simulink model "Arranque_2M"  (R2018b)
settings: Solver=VariableStepAuto  StartTime=0.0  StopTime=32  MaxStep=1e-4  RelTol=1e-3
libraries: powerlib x24, powerlib_meascontrol x12
settings Model: Creator=Guille2  LastModifiedBy=grbos
settings SFSimCC: SimUseLocalCustomCode=off
settings RTWCC: RTWUseLocalCustomCode=off

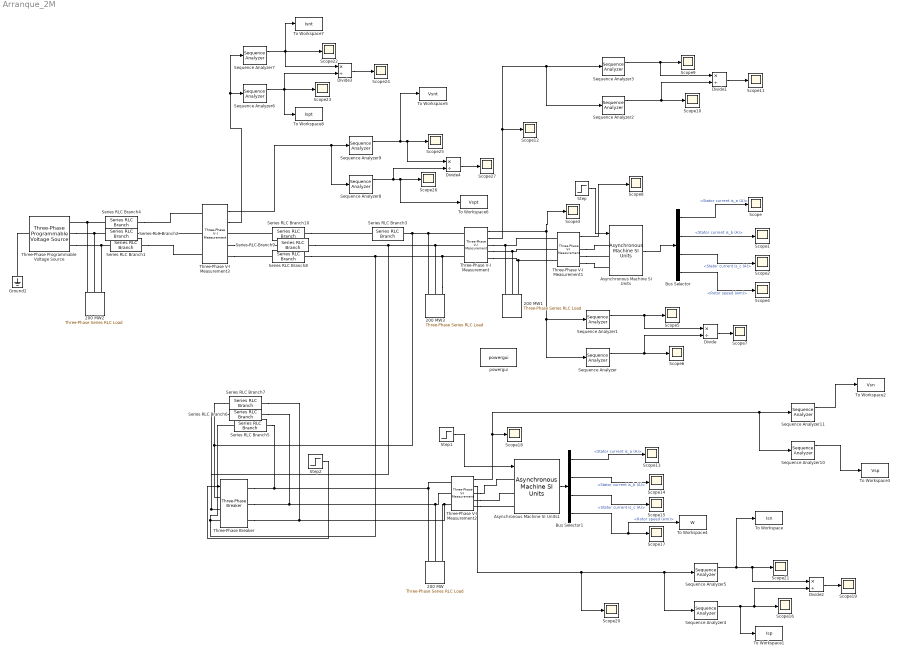
== system Arranque_2M ==
  200 MW{,1..3} (4 alike) : powerlib/Elements/Three-Phase Series RLC Load  LConnTagsString=A|B|C  Configuration=Y (grounded)  NominalVoltage=380  Vabc=[1e3 1e3 1e3]  Vabcp=[1e3 1e3 1e3]  NominalFrequency=50  UnbalancedPower=off  ActivePower=2  InductivePower=0  CapacitivePower=0  Pabc=[10e3 9e3 11e3]  QLabc=[100 90 110]  QCabc=[100 90 110]  Pabcp=[10e3 9e3 11e3]  QLabcp=[100 90 110]  QCabcp=[100 90 110]  Measurements=None  LoadType=constant Z
      settings: SourceProductName=Simscape Electrical
  Asynchronous Machine SI Units : powerlib/Machines/Asynchronous Machine SI Units  RotorType=Squirrel-cage  PresetModel=No  MechanicalLoad=Torque Tm  ShowDetailedParameters=on  ReferenceFrame=Stationary  Units=SI  MeasurementBus=off  NominalParameters=[1.6e+05 400 50]  Stator=[0.01379 0.000152]  Rotor=[0.01728 0.000252]  Cage1=[0.4155 0.002066]  Cage2=[0.4168 0.0003495]  Lm=0.00769  Mechanical=[10 0.05658 1]  PolePairs=2  InitialConditions=[1 0 0 0 0 0 0 0]  SimulateSaturation=off  Saturation=[14.03593122, 27.81365428, 53.79336849, 72.68890987, 97.98006896, 148.6815601, 215.7428561, 302.9841135, 428.7778367 ; 230, 322, 414, 460, 506, 552, 598, 644, 690]  LoadFlowParameters=1492000  TsPowergui=0  TsBlock=-1  IterativeModel=Trapezoidal non iterative  IterativeDiscreteModel=Trapezoidal non iterative  Pmec=1.492e+006
      settings: SourceProductName=Simscape Electrical
  Asynchronous Machine SI Units1 : powerlib/Machines/Asynchronous Machine SI Units  RotorType=Squirrel-cage  PresetModel=No  MechanicalLoad=Torque Tm  ShowDetailedParameters=on  ReferenceFrame=Stationary  Units=SI  MeasurementBus=off  NominalParameters=[1.6e+05 400 50]  Stator=[0.01379 0.000152]  Rotor=[0.01728 0.000252]  Cage1=[0.4155 0.002066]  Cage2=[0.4168 0.0003495]  Lm=0.00769  Mechanical=[10 0.05658 1]  PolePairs=2  InitialConditions=[1 0 0 0 0 0 0 0]  SimulateSaturation=off  Saturation=[14.03593122, 27.81365428, 53.79336849, 72.68890987, 97.98006896, 148.6815601, 215.7428561, 302.9841135, 428.7778367 ; 230, 322, 414, 460, 506, 552, 598, 644, 690]  LoadFlowParameters=1492000  TsPowergui=0  TsBlock=-1  IterativeModel=Trapezoidal non iterative  IterativeDiscreteModel=Trapezoidal non iterative  Pmec=1.492e+006
      settings: SourceProductName=Simscape Electrical
  Bus Selector : BusSelector  OutputSignals=Stator measurements.Stator current is_a (A),Stator measurements.Stator current is_b (A),Stator measurements.Stator current is_c (A),Mechanical.Rotor speed (wm)
  Bus Selector1 : BusSelector  OutputSignals=Stator measurements.Stator current is_a (A),Stator measurements.Stator current is_b (A),Stator measurements.Stator current is_c (A),Mechanical.Rotor speed (wm)
  Divide{,1..4} (5 alike) : Product  Inputs=*/
  Ground2 : powerlib/Elements/Ground  LConnTagsString=a
      settings: SourceProductName=Simscape Electrical
  Scope{,1..27} (28 alike) : Scope
  Sequence Analyzer{,2,4,6,8,10} (6 alike) : powerlib_meascontrol/Measurements/Sequence Analyzer  Freq=50  n=1  seq=Positive  InInit=[1, 0]  Ts=0
      settings: SourceProductName=Simscape Electrical  SourceProductBaseCode=PS
  Sequence Analyzer{1,3,5,7,9,11} (6 alike) : powerlib_meascontrol/Measurements/Sequence Analyzer  Freq=50  n=1  seq=Negative  InInit=[1, 0]  Ts=0
      settings: SourceProductName=Simscape Electrical  SourceProductBaseCode=PS
  Series RLC Branch{1..4} (4 alike) : powerlib/Elements/Series RLC Branch  LConnTagsString=__new0  RConnTagsString=__new0  BranchType=R  Resistance=0.01  Inductance=1.0  SetiL0=off  InitialCurrent=0  Capacitance=1.0  Setx0=off  InitialVoltage=0  Measurements=None
      settings: SourceProductName=Simscape Electrical
  Series RLC Branch10 : powerlib/Elements/Series RLC Branch  LConnTagsString=__new0  RConnTagsString=__new0  BranchType=R  Resistance=0.02  Inductance=1.0  SetiL0=off  InitialCurrent=0  Capacitance=1.0  Setx0=off  InitialVoltage=0  Measurements=None
      settings: SourceProductName=Simscape Electrical
  Series RLC Branch5 : powerlib/Elements/Series RLC Branch  LConnTagsString=__new0  RConnTagsString=__new0  BranchType=R  Resistance=300  Inductance=1.0  SetiL0=off  InitialCurrent=0  Capacitance=1.0  Setx0=off  InitialVoltage=0  Measurements=None
      settings: SourceProductName=Simscape Electrical
  Series RLC Branch6 : powerlib/Elements/Series RLC Branch  LConnTagsString=__new0  RConnTagsString=__new0  BranchType=R  Resistance=300  Inductance=1.0  SetiL0=off  InitialCurrent=0  Capacitance=1.0  Setx0=off  InitialVoltage=0  Measurements=None
      settings: SourceProductName=Simscape Electrical
  Series RLC Branch7 : powerlib/Elements/Series RLC Branch  LConnTagsString=__new0  RConnTagsString=__new0  BranchType=R  Resistance=300  Inductance=1.0  SetiL0=off  InitialCurrent=0  Capacitance=1.0  Setx0=off  InitialVoltage=0  Measurements=None
      settings: SourceProductName=Simscape Electrical
  Series RLC Branch8 : powerlib/Elements/Series RLC Branch  LConnTagsString=__new0  RConnTagsString=__new0  BranchType=R  Resistance=0.02  Inductance=1.0  SetiL0=off  InitialCurrent=0  Capacitance=1.0  Setx0=off  InitialVoltage=0  Measurements=None
      settings: SourceProductName=Simscape Electrical
  Series RLC Branch9 : powerlib/Elements/Series RLC Branch  LConnTagsString=__new0  RConnTagsString=__new0  BranchType=R  Resistance=0.02  Inductance=1.0  SetiL0=off  InitialCurrent=0  Capacitance=1.0  Setx0=off  InitialVoltage=0  Measurements=None
      settings: SourceProductName=Simscape Electrical
  Step : Step  Time=8  After=500  SampleTime=0
  Step1 : Step  Time=24  After=500  SampleTime=0
  Step2 : Step  Time=16  SampleTime=0
  Three-Phase Programmable Voltage Source : powerlib/Electrical Sources/Three-Phase Programmable Voltage Source  PositiveSequence="[380  0 50]"  VariationEntity=None  VariationType=Table of time-amplitude pairs  VariationTypeAlt=Step  VariationStep=0.5  VariationRate=10  VariationMagnitude=0.3  VariationFrequency=2  VariationTiming=[1 2]  VariationPhaseA=off  Amplitudes=[1 0.8 1.2 1.0]  TimeValues=[0 0.1 0.15 0.2]  HarmonicGeneration=off  HarmonicA=[1 0.73 0 1]  HarmonicB=[0 0 0 0]  Timing="[8  16]"  BusType=swing  Pref=0  Qref=0  Qmin=-inf  Qmax=inf
      settings: SourceProductName=Simscape Electrical
  Three-Phase V-I Measurement : powerlib/Measurements/Three-Phase V-I Measurement  VoltageMeasurement=phase-to-ground  SetLabelV=off  LabelV=Vabc  Vpu=off  VpuLL=off  CurrentMeasurement=yes  SetLabelI=off  LabelI=Iabc  Ipu=off  Pbase=100e6  Vbase=500e3  OutputType=Complex  PhasorSimulation=off  PSBequivalent=0
      settings: SourceProductName=Simscape Electrical
  Three-Phase V-I Measurement1 : powerlib/Measurements/Three-Phase V-I Measurement  VoltageMeasurement=phase-to-phase  SetLabelV=off  LabelV=Vabc  Vpu=off  VpuLL=off  CurrentMeasurement=yes  SetLabelI=off  LabelI=Iabc  Ipu=off  Pbase=100e6  Vbase=500e3  OutputType=Complex  PhasorSimulation=off  PSBequivalent=0
      settings: SourceProductName=Simscape Electrical
  Three-Phase V-I Measurement2 : powerlib/Measurements/Three-Phase V-I Measurement  VoltageMeasurement=phase-to-ground  SetLabelV=off  LabelV=Vabc  Vpu=off  VpuLL=off  CurrentMeasurement=yes  SetLabelI=off  LabelI=Iabc  Ipu=off  Pbase=100e6  Vbase=500e3  OutputType=Complex  PhasorSimulation=off  PSBequivalent=0
      settings: SourceProductName=Simscape Electrical
  Three-Phase V-I Measurement3 : powerlib/Measurements/Three-Phase V-I Measurement  VoltageMeasurement=phase-to-ground  SetLabelV=off  LabelV=Vabc  Vpu=off  VpuLL=off  CurrentMeasurement=yes  SetLabelI=off  LabelI=Iabc  Ipu=off  Pbase=100e6  Vbase=500e3  OutputType=Complex  PhasorSimulation=off  PSBequivalent=0
      settings: SourceProductName=Simscape Electrical
  Three-Phase Breaker : powerlib/Elements/Three-Phase Breaker  InitialState=open  SwitchA=on  SwitchB=on  SwitchC=on  SwitchTimes="[1/60  5/60]"  External=on  BreakerResistance=0.0001  SnubberResistance=inf  SnubberCapacitance=inf  Measurements=None
      settings: SourceProductName=Simscape Electrical
  To Workspace : ToWorkspace  VariableName=Isn  SaveFormat=Timeseries  SampleTime=0.001
  To Workspace1 : ToWorkspace  VariableName=Isp  SaveFormat=Timeseries  SampleTime=0.001
  To Workspace2 : ToWorkspace  VariableName=Vsn  SaveFormat=Timeseries  SampleTime=0.001
  To Workspace3 : ToWorkspace  VariableName=Vsp  SaveFormat=Timeseries  SampleTime=0.001
  To Workspace4 : ToWorkspace  VariableName=W  SaveFormat=Timeseries  SampleTime=0.001
  To Workspace5 : ToWorkspace  VariableName=Vsnt  SaveFormat=Timeseries  SampleTime=0.001
  To Workspace6 : ToWorkspace  VariableName=Vspt  SaveFormat=Timeseries  SampleTime=0.001
  To Workspace7 : ToWorkspace  VariableName=Isnt  SaveFormat=Timeseries  SampleTime=0.001
  To Workspace8 : ToWorkspace  VariableName=Ispt  SaveFormat=Timeseries  SampleTime=0.001
  powergui : powerlib/powergui  Priority=1  SimulationMode=Continuous  SampleTime=50e-6  frequency=60  Iterations=50  frequencyindice=50  Pbase=100e6  ErrMax=1e-4  UnitsV=kV  UnitsW=MW  buscounter=0  FunctionMessages=off  echomessages=off  EnableUseOfTLC=off  CurrentSourceSwitches=off  DisableSnubberDevices=off  DisableRonSwitches=off  DisableVfSwitches=off  DisplayEquations=off  SolverType=Tustin/Backward Euler (TBE)  Interpol=off  ExternalGateDelay=off  methode=off  Ts=100  x0status=blocks  SPID=on  SwTol=0  HookPort=off  RestoreLinks=warning  ResistiveCurrentMeasurement=off  Frange=[0:2:500]  Ylog=off  Xlog=on  ShowGrid=off  save=off  variable=ZData  structure=0  ZoomFFT=off  StartTime=0.0  cycles=1  DisplayStyle=1  fundamental=60  FreqAxis=off  MaxFrequency=1000  frequencyindicesteady=1  RmsSteady=1  display=off
      settings: SourceProductName=Simscape Electrical
  wires:
  Bus Selector/3 -> Scope2/1  "<Stator current is_c (A)>"
  Bus Selector/4 -> Scope4/1  "<Rotor speed (wm)>"
  Bus Selector/2 -> Scope1/1  "<Stator current is_b (A)>"
  Asynchronous Machine SI Units/1 -> Bus Selector/1
  Bus Selector/1 -> Scope/1  "<Stator current is_a (A)>"
  Step/1 -> Asynchronous Machine SI Units/1
  Three-Phase V-I Measurement/1 -> Scope3/1, Sequence Analyzer/1, Sequence Analyzer1/1
  Sequence Analyzer/1 -> Scope6/1, Divide/2
  Sequence Analyzer1/1 -> Divide/1, Scope5/1
  Divide/1 -> Scope7/1
  Three-Phase V-I Measurement1/1 -> Scope8/1
  Divide1/1 -> Scope11/1
  Sequence Analyzer3/1 -> Divide1/1, Scope9/1
  Sequence Analyzer2/1 -> Scope10/1, Divide1/2
  Three-Phase V-I Measurement/2 -> Scope12/1, Sequence Analyzer2/1, Sequence Analyzer3/1
  Asynchronous Machine SI Units1/1 -> Bus Selector1/1
  Bus Selector1/3 -> Scope15/1  "<Stator current is_c (A)>"
  Bus Selector1/4 -> To Workspace4/1, Scope17/1  "<Rotor speed (wm)>"
  Bus Selector1/1 -> Scope13/1  "<Stator current is_a (A)>"
  Step1/1 -> Asynchronous Machine SI Units1/1
  Bus Selector1/2 -> Scope14/1  "<Stator current is_b (A)>"
  Step2/1 -> Three-Phase Breaker/1
  Sequence Analyzer4/1 -> Scope16/1, Divide2/2, To Workspace1/1
  Divide2/1 -> Scope19/1
  Sequence Analyzer5/1 -> To Workspace/1, Divide2/1, Scope21/1
  Three-Phase V-I Measurement2/2 -> Scope20/1, Sequence Analyzer4/1, Sequence Analyzer5/1
  Three-Phase V-I Measurement3/2 -> Sequence Analyzer6/1, Sequence Analyzer7/1
  Divide3/1 -> Scope24/1
  Sequence Analyzer7/1 -> Scope22/1, Divide3/1, To Workspace7/1
  Sequence Analyzer6/1 -> Scope23/1, To Workspace8/1, Divide3/2
  Three-Phase V-I Measurement3/1 -> Sequence Analyzer8/1, Sequence Analyzer9/1
  Sequence Analyzer8/1 -> To Workspace6/1, Scope26/1, Divide4/2
  Sequence Analyzer9/1 -> To Workspace5/1, Divide4/1, Scope25/1
  Divide4/1 -> Scope27/1
  Three-Phase V-I Measurement2/1 -> Sequence Analyzer10/1, Sequence Analyzer11/1, Scope18/1
  Sequence Analyzer11/1 -> To Workspace2/1
  Sequence Analyzer10/1 -> To Workspace3/1
  connections:
  Ground2/LConn1 -- Three-Phase Programmable Voltage Source/LConn1
  Series RLC Branch10/RConn1 -- Series RLC Branch3/LConn1
  Three-Phase Programmable Voltage Source/RConn2 -- Series RLC Branch2/LConn1 -- 200 MW2/LConn2
  Three-Phase Programmable Voltage Source/RConn3 -- Series RLC Branch1/LConn1 -- 200 MW2/LConn3
  Three-Phase V-I Measurement/RConn1 -- 200 MW1/LConn1 -- Three-Phase V-I Measurement1/LConn1
  Three-Phase V-I Measurement/RConn2 -- 200 MW1/LConn2 -- Three-Phase V-I Measurement1/LConn2
  Three-Phase V-I Measurement/RConn3 -- 200 MW1/LConn3 -- Three-Phase V-I Measurement1/LConn3
  Three-Phase V-I Measurement1/RConn1 -- Asynchronous Machine SI Units/LConn1
  Three-Phase V-I Measurement1/RConn2 -- Asynchronous Machine SI Units/LConn2
  Three-Phase V-I Measurement1/RConn3 -- Asynchronous Machine SI Units/LConn3
  200 MW3/LConn3 -- Three-Phase V-I Measurement/LConn3 -- Series RLC Branch8/RConn1 -- Series RLC Branch5/LConn1 -- Three-Phase Breaker/LConn3
  Series RLC Branch6/LConn1 -- Three-Phase V-I Measurement/LConn2 -- 200 MW3/LConn2 -- Series RLC Branch9/RConn1 -- Three-Phase Breaker/LConn2
  Series RLC Branch4/LConn1 -- 200 MW2/LConn1 -- Three-Phase Programmable Voltage Source/RConn1
  Three-Phase V-I Measurement2/RConn2 -- Asynchronous Machine SI Units1/LConn2
  Three-Phase V-I Measurement2/RConn3 -- Asynchronous Machine SI Units1/LConn3
  Three-Phase V-I Measurement2/RConn1 -- Asynchronous Machine SI Units1/LConn1
  Three-Phase Breaker/RConn2 -- Series RLC Branch6/RConn1 -- Three-Phase V-I Measurement2/LConn2 -- 200 MW/LConn2
  Three-Phase Breaker/RConn1 -- Series RLC Branch5/RConn1 -- Three-Phase V-I Measurement2/LConn1 -- 200 MW/LConn1
  Three-Phase Breaker/RConn3 -- Series RLC Branch7/RConn1 -- 200 MW/LConn3 -- Three-Phase V-I Measurement2/LConn3
  Series RLC Branch4/RConn1 -- Three-Phase V-I Measurement3/LConn1
  Series RLC Branch2/RConn1 -- Three-Phase V-I Measurement3/LConn2
  Series RLC Branch1/RConn1 -- Three-Phase V-I Measurement3/LConn3
  Series RLC Branch10/LConn1 -- Three-Phase V-I Measurement3/RConn1
  Three-Phase V-I Measurement3/RConn2 -- Series RLC Branch9/LConn1
  Three-Phase V-I Measurement3/RConn3 -- Series RLC Branch8/LConn1
  Three-Phase Breaker/LConn1 -- Three-Phase V-I Measurement/LConn1 -- 200 MW3/LConn1 -- Series RLC Branch3/RConn1 -- Series RLC Branch7/LConn1
